simulink model "Quadcopter_Dynamics"  (R2021a)
settings: Solver=VariableStepAuto  StartTime=0.0  StopTime=10.0  RelTol=1e-3
settings Model: Creator=Hameed  LastModifiedBy=Hameed

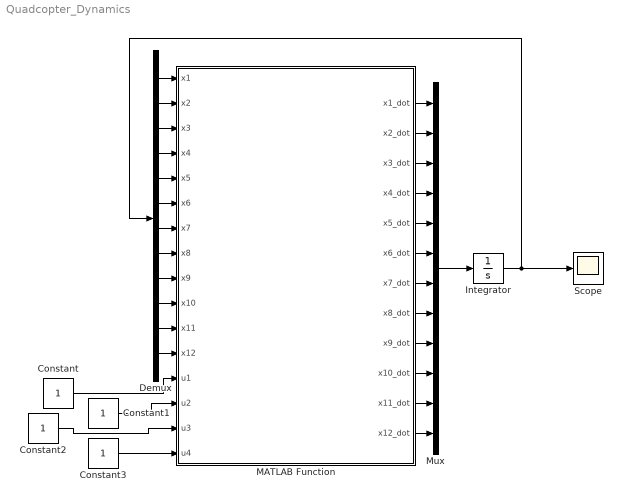
== system Quadcopter_Dynamics ==
  Constant{,1..3} (4 alike) : Constant
  Demux : Demux  Outputs=12
  Integrator : Integrator  InitialCondition=[0;0;0;0;0;0;0;0;0;0;0;0]
  MATLAB Function : MATLAB Function  TreatAsAtomicUnit=on
  Mux : Mux  Inputs=12
  Scope : Scope
  wires:
  MATLAB Function/1(x1_dot) -> Mux/1
  MATLAB Function/2(x2_dot) -> Mux/2
  MATLAB Function/3(x3_dot) -> Mux/3
  MATLAB Function/4(x4_dot) -> Mux/4
  MATLAB Function/5(x5_dot) -> Mux/5
  MATLAB Function/6(x6_dot) -> Mux/6
  MATLAB Function/7(x7_dot) -> Mux/7
  MATLAB Function/8(x8_dot) -> Mux/8
  MATLAB Function/9(x9_dot) -> Mux/9
  MATLAB Function/10(x10_dot) -> Mux/10
  MATLAB Function/11(x11_dot) -> Mux/11
  MATLAB Function/12(x12_dot) -> Mux/12
  Mux/1 -> Integrator/1
  Demux/1 -> MATLAB Function/1(x1)
  Demux/2 -> MATLAB Function/2(x2)
  Demux/3 -> MATLAB Function/3(x3)
  Demux/4 -> MATLAB Function/4(x4)
  Demux/5 -> MATLAB Function/5(x5)
  Demux/6 -> MATLAB Function/6(x6)
  Demux/7 -> MATLAB Function/7(x7)
  Demux/8 -> MATLAB Function/8(x8)
  Demux/9 -> MATLAB Function/9(x9)
  Demux/10 -> MATLAB Function/10(x10)
  Demux/11 -> MATLAB Function/11(x11)
  Demux/12 -> MATLAB Function/12(x12)
  Integrator/1 -> Demux/1, Scope/1
  Constant3/1 -> MATLAB Function/16(u4)
  Constant2/1 -> MATLAB Function/15(u3)
  Constant1/1 -> MATLAB Function/14(u2)
  Constant/1 -> MATLAB Function/13(u1)

== matlab function Quadcopter_Dynamics/MATLAB Function ==
  data: x1 input; x1_dot output; x2 input; x3 input; x4 input; x5 input; x6 input; x7 input; x8 input; x9 input; x10 input; x11 input; x12 input; u1 input; u2 input; u3 input; u4 input; x2_dot output; x3_dot output; x4_dot output; x5_dot output; x6_dot output; x7_dot output; x8_dot output; x9_dot output; x10_dot output; x11_dot output; x12_dot output
function [x1_dot,x2_dot,x3_dot,x4_dot,x5_dot,x6_dot,x7_dot,x8_dot,x9_dot,x10_dot,x11_dot,x12_dot]= fcn(x1,x2,x3,x4,x5,x6,x7,x8,x9,x10,x11,x12,u1,u2,u3,u4)
% x=x1;
% y=x2,
% z=x3
% phi=x4;
% theta=x5;
% sai=x6;
% x_dot=x7;
% y_dot=x8,
% z_dot=x9
% phi_dot=x10;
% theta_dot=x11;
% sai_dot=x12;

Ixx= 1.2; 
Iyy= 1.2;
Izz= 2.3;
k= 1;
l= 0.25;
m= 2;
b= 0.2;
g= 9.81;

T = k*(u1+u2+u3+u4);
x789= -g*[0;0;1]+(T/m)*[sin(x6)*sin(x5)*sin(x4)+sin(x6)*sin(x4);cos(x6)*cos(x5)*cos(x4)-cos(x6)*cos(x4);cos(x5)*cos(x4)];

tB= [l*k*(-u2 + u4);l*k*(-u1 + u3);b*(-u1+u2-u3+u4)];


C11=0
C12=(Iyy-Izz)*(x7*cos(x4)*sin(x4)+x12*sin(x4)^2*cos(x5))+(Izz-Iyy)*x12*cos(x4)^2*cos(x5)-Ixx*x12*cos(x5);
C13=(Izz-Iyy)*(x12*cos(x4)*sin(x4)*cos(x5)^2);
C21=(Izz-Iyy)*(x7*cos(x4)*sin(x4)+x12*sin(x4)*cos(x5))+(Iyy-Izz)*x12*cos(x4)^2*cos(x5)-Ixx*x12*cos(x5);
C22=(Izz-Iyy)*x10*cos(x4)*sin(x4);
C23= -Ixx*x12*sin(x5)*cos(x5)+Iyy*x12*sin(x4)^2*sin(x5)*cos(x5)+ Izz*x12*cos(x4)^2*sin(x5)*cos(x5);
C31=(Iyy-Izz)*(x12*cos(x5)^2*sin(x4)*cos(x4))-Ixx*x11*cos(x5);
C32= (Izz-Iyy)*(x11*cos(x4)*sin(x4)*sin(x5)+x10*sin(x4)^2*cos(x5))+(Iyy-Izz)*x10*cos(x4)^2*cos(x5)+Ixx*x12*cos(x5)*cos(x5)-Iyy*x12*sin(x10)^2*sin(x5)*cos(x5)-Izz*x12*cos(x10)^2*sin(x5)*cos(x5);
C33=(Iyy-Izz)*x10*cos(x4)*sin(x4)*cos(x5)^2-Iyy*x11*sin(x4)^2*cos(x5)*sin(x5)-Izz*x11*cos(x4)^2*cos(x5)*sin(x5)+Ixx*x11*cos(x5)*sin(x5);
Cnndot=[C11 C12 C13;C21 C22 C23;C31 C32 C33];

%ndot=[x10_dot;x11_dot;x12_dot];
ndot=[x10;x11;x12];


W = [1, 0, -sin(x5);
    0, cos(x4), cos(x5)*sin(x4);
    0, -sin(x4), cos(x5)*cos(x4)];
I = [Ixx,0,0;0,Iyy,0;0,0,Izz];
J = W.'*I*W;

x101112= inv(J)*(tB-Cnndot*ndot);

x1_dot=x7;
x2_dot=x8;
x3_dot=x9;
x4_dot=x10;
x5_dot=x11;
x6_dot=x12;
x7_dot=x789(1);
x8_dot=x789(2);
x9_dot=x789(3);
x10_dot=x101112(1);
x11_dot=x101112(2);
x12_dot=x101112(3);


%y=u;
